simulink model "quad_state_no_sensor_noise"  (R2021a)
settings: Solver=FixedStepAuto  StartTime=0.0  StopTime=10.0  RelTol=1e-3
undefined symbols (not defined in the file): sim_freq
settings Model: Creator=francois  LastModifiedBy=esl
settings SolverCC: AlgebraicLoopSolver=TrustRegion
settings DebuggingCC: SFMachineParentedDataDiag=warning

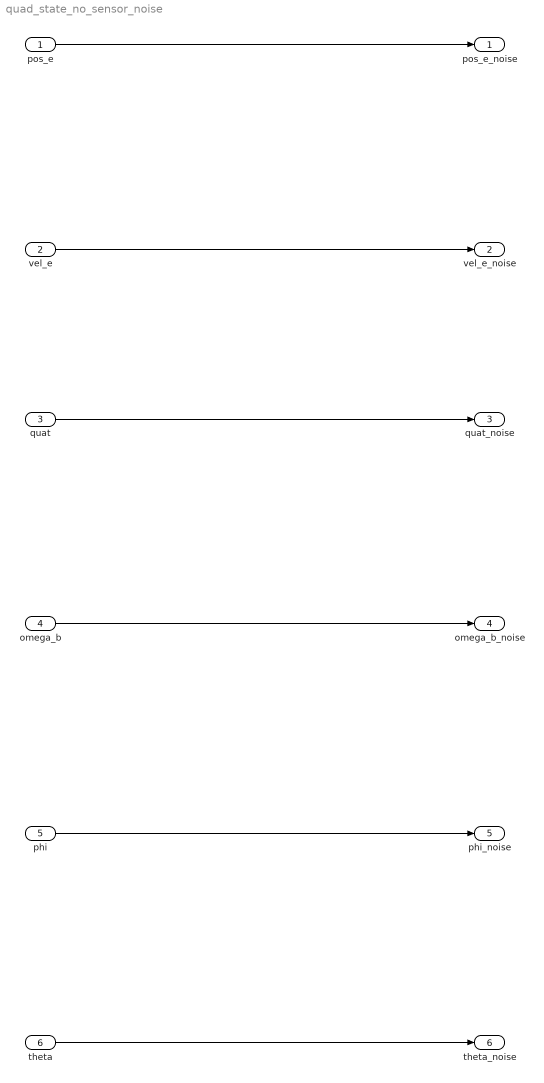
== system quad_state_no_sensor_noise ==
  pos_e : Inport  PortDimensions=3  SampleTime=1/sim_freq
  vel_e : Inport  Port=2  PortDimensions=3  SampleTime=1/sim_freq
  quat : Inport  Port=3  PortDimensions=4  SampleTime=1/sim_freq
  omega_b : Inport  Port=4  PortDimensions=3  SampleTime=1/sim_freq
  phi : Inport  Port=5  PortDimensions=1  SampleTime=1/sim_freq
  theta : Inport  Port=6  PortDimensions=1  SampleTime=1/sim_freq
  pos_e_noise : Outport  PortDimensions=3  VectorParamsAs1DForOutWhenUnconnected=off
  vel_e_noise : Outport  Port=2  PortDimensions=3  VectorParamsAs1DForOutWhenUnconnected=off
  quat_noise : Outport  Port=3  PortDimensions=4  VectorParamsAs1DForOutWhenUnconnected=off
  omega_b_noise : Outport  Port=4  PortDimensions=3  VectorParamsAs1DForOutWhenUnconnected=off
  phi_noise : Outport  Port=5  VectorParamsAs1DForOutWhenUnconnected=off
  theta_noise : Outport  Port=6  VectorParamsAs1DForOutWhenUnconnected=off
  wires:
  quat/1 -> quat_noise/1
  vel_e/1 -> vel_e_noise/1
  omega_b/1 -> omega_b_noise/1
  pos_e/1 -> pos_e_noise/1
  phi/1 -> phi_noise/1
  theta/1 -> theta_noise/1
